simulink library "sm_rollerV_lib_lower_frame_r9"  (R2026a)
settings: Solver=VariableStepAuto
undefined symbols (not defined in the file): Excv, Left, Right
libraries: sm_rollerV_lib_underc_elem x2, sm_rollerV_lib_underc_i1u2l7 x2
Description:
  | Copyright 2023-2026 The MathWorks, Inc.
settings Model: Creator=smiller  LastModifiedBy=smiller

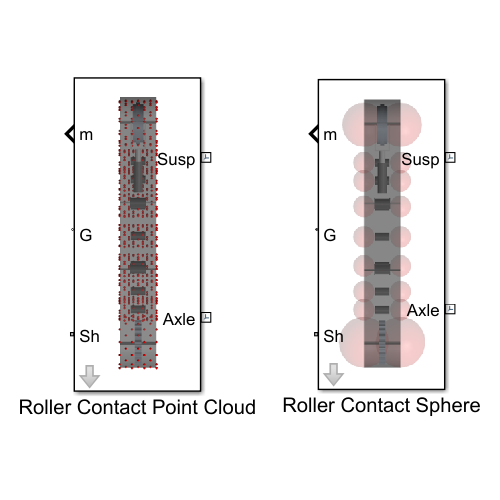
[thumbnail: Simulink's stored preview of the top-level diagram]
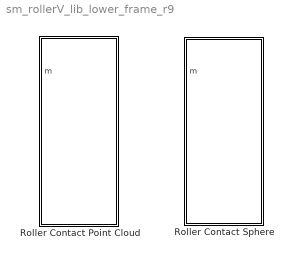
== system sm_rollerV_lib_lower_frame_r9 ==
  Roller Contact Point Cloud : Subsystem  mask(Lower Frame with Roller Point Cloud Contact Geometry){popup_leftOrRight=Left, sprk_xc=Excv.Sprocket.sprocket_xc, sprk_len=Excv.Sprocket.sprk_width, sprk_rho=Excv.Sprocket.density, sprk_clr=Excv.Sprocket.clr, sprk_opc=Excv.Sprocket.opc, sprk_contact_geo_ptcld=Excv.Sprocket.ground_contact.ptcld.pts, sprk_contact_geo_rad=Excv.Sprocket.ground_contact.ptcld.rad, sprk_contact_geo_clr=Excv.Sprocket.ground_contact.ptcld.clr, sprk_contact_geo_opc=Excv.Sprocket.ground_contact.ptcld.opc, idler_rad=Excv.Idler.rad, idler_len=Excv.Idler.len, idler_rho=Excv.Idler.rho, idler_clr=Excv.Idler.clr, idler_opc=Excv.Idler.opc, idler_contact_geo_ptcld=Excv.Idler.ground_contact.ptcld.pts, idler_contact_geo_rad=Excv.Idler.ground_contact.ptcld.rad, idler_contact_geo_clr=Excv.Idler.ground_contact.ptcld.clr, idler_contact_geo_opc=Excv.Idler.ground_contact.ptcld.opc, roller_upper_rad=Excv.Roller.Upper.rad, roller_upper_len=Excv.Roller.Upper.len, roller_upper_rho=Excv.Roller.Upper.rho, roller_upper_clr=Excv.Roller.Upper.clr, roller_upper_opc=Excv.Roller.Upper.opc, roller_upper_contgeo_clr=[1.0 0.0 0.0], roller_upper_contgeo_opc=1, roller_lower_rad=Excv.Roller.Lower.rad, roller_lower_len=Excv.Roller.Lower.len, roller_lower_rho=Excv.Roller.Lower.rho, roller_lower_clr=Excv.Roller.Lower.clr, roller_lower_opc=Excv.Roller.Lower.opc, roller_lower_contgeo_ptcld=Excv.Roller.Lower.ground_contact.ptcld.pts, roller_lower_contgeo_rad=Excv.Roller.Lower.ground_contact.ptcld.rad, roller_lower_contgeo_clr=Excv.Roller.Lower.ground_contact.ptcld.clr, roller_lower_contgeo_opc=Excv.Roller.Lower.ground_contact.ptcld.opc, tensioner_cyl_len=Excv.Idler.Tensioner.cyl.len, tensioner_cyl_rad=Excv.Idler.Tensioner.cyl.rad, tensioner_cyl_rho=Excv.Idler.Tensioner.cyl.rho, tensioner_cyl_clr=Excv.Idler.Tensioner.cyl.clr, tensioner_cyl_opc=Excv.Idler.Tensioner.cyl.opc, tensioner_pist_len=Excv.Idler.Tensioner.piston.len, tensioner_pist_rad=Excv.Idler.Tensioner.piston.rad, tensioner_pist_rho=Excv.Idler.Tensioner.piston.rho, tensioner_pist_clr=Excv.Idler.Tensioner.piston.clr, tensioner_pist_opc=Excv.Idler.Tensioner.piston.opc, tensioner_br_length=Excv.Idler.Tensioner.bracket.len, tensioner_br_width=Excv.Idler.Tensioner.bracket.wid, tensioner_br_height=Excv.Idler.Tensioner.bracket.height, tensioner_br_thk=Excv.Idler.Tensioner.bracket.thk, tensioner_br_rho=Excv.Idler.Tensioner.bracket.rho, tensioner_br_clr=Excv.Idler.Tensioner.bracket.clr, tensioner_br_opc=Excv.Idler.Tensioner.bracket.opc, idler_max_ext=Excv.Idler.Tensioner.cyl.max_ext, sprk_rolling_rad=Excv.Sprocket.ground_contact.rolling_radius, idler_rolling_rad=Excv.Idler.ground_contact.rolling_radius, roller_lower_rolling_rad=Excv.Roller.Lower.ground_contact.rolling_radius, lext=1e-3, track_w=Excv.Shoe.w, sprocket_cyl_clr=Excv.Sprocket.clr, sprocket_cyl_opc=1, idler_cyl_clr=Excv.Idler.clr, idler_cyl_opc=1, roller_cyl_clr=Excv.Roller.Lower.clr, roller_cyl_opc=1, accMn=0.65, accMx=0.75, acc_clr=[0.8 0.8 0.8], acc_opc=1, roller_upper_x=Excv.Frame.Sprk2UpperX, roller_lower_x=Excv.Frame.Sprk2LowerX, idler_x=Excv.Frame.IdlerAssyX, axle_x=Excv.Frame.AxleX, roller_upper_y=Excv.Frame.Sprk2UpperY, roller_lower_y=Excv.Frame.Sprk2LowerY, idler_y=Excv.Frame.Sprk2IdlerY, axle_y=Excv.Frame.AxleY, frame_cg_offset=Excv.Frame.CGOffset, frame_mass=Excv.Frame.Mass, frame_moi=Excv.Frame.MOI, frame_poi=Excv.Frame.POI, frame_susp_offset=Excv.Frame.SuspOffset, track_m=Excv.Vis.Track.m, track_cg_offset=Excv.Vis.Track.cg, track_moi=Excv.Vis.Track.moi, track_poi=Excv.Vis.Track.poi, track_xc=Excv.Vis.Track.track_xc, track_clr=Excv.Vis.Track.clr, track_opc=Excv.Vis.Track.opc, popup_sense_roller=Constraint Force}
      mask prompts: popup_leftOrRight "Left or Right"; sprk_xc "Extrusion Data [x y] (m)"; sprk_len "Length (m)"; sprk_rho "Density (kg/m^3)"; sprk_clr "Color [R G B] (0-1)"; sprk_opc "Opacity (0-1)"; sprk_contact_geo_ptcld "Point Cloud Data [x y z] (m)"; sprk_contact_geo_rad "Radius (m)"; sprk_contact_geo_clr "Color [R G B] (0-1)"; sprk_contact_geo_opc "Opacity (0-1)"; idler_rad "Idler Radius (m)"; idler_len "Length (m)"; idler_rho "Density (kg/m^3)"; idler_clr "Color [R G B] (0-1)"; idler_opc "Opacity (0-1)"; idler_contact_geo_ptcld "Point Cloud Data [x y z] (m)"; idler_contact_geo_rad "Point Radius (m)"; idler_contact_geo_clr "Color [R G B] (0-1)"; idler_contact_geo_opc "Opacity (0-1)"; roller_upper_rad "Radius (m)"; roller_upper_len "Length (m)"; roller_upper_rho "Density (kg/m^3)"; roller_upper_clr "Color [R G B] (0-1)"; roller_upper_opc "Opacity (0-1)"; roller_upper_contgeo_clr "Color [R G B] (0-1)"; roller_upper_contgeo_opc "Opacity (0-1)"; roller_lower_rad "Lower Roller Radius (m)"; roller_lower_len "Length (m)"; roller_lower_rho "Density (kg/m^3)"; roller_lower_clr "Color [R G B] (0-1)"; roller_lower_opc "Opacity (0-1)"; roller_lower_contgeo_ptcld "Point Cloud [x y z] (m)"; roller_lower_contgeo_rad "Point Radius (m)"; roller_lower_contgeo_clr "Color [R G B] (0-1)"; roller_lower_contgeo_opc "Opacity (0-1)"; tensioner_cyl_len "Length (m)"; tensioner_cyl_rad "Radius (m)"; tensioner_cyl_rho "Density (kg/m^3)"; tensioner_cyl_clr "Color [R G B] (0-1)"; tensioner_cyl_opc "Opacity (0-1)"; tensioner_pist_len "Length (m)"; tensioner_pist_rad "Radius (m)"; tensioner_pist_rho "Density (kg/m^3)"; tensioner_pist_clr "Color [R G B] (0-1)"; tensioner_pist_opc "Opacity (0.1)"; tensioner_br_length "Length (m)"; tensioner_br_width "Width (m)"; tensioner_br_height "Height (m)"; tensioner_br_thk "Thickness (m)"; tensioner_br_rho "Density (kg/m^3)"; tensioner_br_clr "Color [R G B] (0-1)"; tensioner_br_opc "Opacity (0-1)"; idler_max_ext "Max Extension in Track (m)"; sprk_rolling_rad "Sprocket Rolling Radius (m)"; idler_rolling_rad "Idler Rolling Radius (m)"; roller_lower_rolling_rad "Lower Roller Rolling Radius (m)"; lext "Length Extensions (m)"; track_w "Shoe Width (m)"; sprocket_cyl_clr "Cylinder Color [R G B] (0-1)"; sprocket_cyl_opc "Cylinder Opacity (0-1)"; idler_cyl_clr "Cylinder Color [R G B] (0-1)"; idler_cyl_opc "Cylinder Opacity (0-1)"; roller_cyl_clr "Cylinder Color [R G B] (0-1)"; roller_cyl_opc "Cylinder Opacity (0-1)"; accMn "Accent Min Radius (0-1)"; accMx "Accent Max Radius (0-1)"; acc_clr "Accent Color [R G B] (0-1)"; acc_opc "Accent Opacity (0-1)"; roller_upper_x "Upper Rollers (vector) (m)"; roller_lower_x "Lower Rollers (vector) (m)"; idler_x "Idler Wheel (m)"; axle_x "Axle Offset (m)"; roller_upper_y "Sprocket to Upper Rollers (m)"; roller_lower_y "Sprocket to Lower Rollers (m)"; idler_y "Sprocket to Idler (m)"; axle_y "Sprocket to Axle (m)"; frame_cg_offset "CG Offset from Sprocket [x y z] (m)"; frame_mass "Mass (kg)"; frame_moi "Moments of Inertia [Ixx Iyy Izz] (kg*m^2)"; frame_poi "Products of Inertia [Ixx Iyy Izz] (kg*m^2)"; frame_susp_offset "Suspension Offset from Sprocket [x y z] (m)"; track_m "Mass"; track_cg_offset "CG Offset from Sprocket Ctr [x y z] (m)"; track_moi "Moments of Inertia  (kg*m^2)"; track_poi "Products of Inertia  (kg*m^2)"; track_xc "Track Visual Extrusion Profile [x y] (m)"; track_clr "Color [R G B] (0-1)"; track_opc "Opacity (0-1)"; popup_sense_roller "Roller"
      mask help: Models an undercarriage with rollers that contact the ground via a point cloud. Includes sprocket, rollers, and idler with tensioner. The sprocket has a 1D rotational mechanical interface to the drivetrain.
      mask init:
      | bh = gcb;
      | set_param([bh '/Undercarriage'],'popup_sense_roller',get_param(bh,'popup_sense_roller'));
      mask TypeOptions popup_leftOrRight: Undercarriage/popup_leftOrRight
      mask TypeOptions sprk_xc: Undercarriage/sprk_xc
      mask TypeOptions sprk_len: Undercarriage/sprk_len
      mask TypeOptions sprk_rho: Undercarriage/sprk_rho
      mask TypeOptions sprk_clr: Undercarriage/sprk_clr
      mask TypeOptions sprk_opc: Undercarriage/sprk_opc
      mask TypeOptions sprk_contact_geo_ptcld: Undercarriage/sprk_contact_geo_ptcld
      mask TypeOptions sprk_contact_geo_rad: Undercarriage/sprk_contact_geo_rad
      mask TypeOptions sprk_contact_geo_clr: Undercarriage/sprk_contact_geo_clr
      mask TypeOptions sprk_contact_geo_opc: Undercarriage/sprk_contact_geo_opc
      mask TypeOptions idler_rad: Undercarriage/idler_rad
      mask TypeOptions idler_len: Undercarriage/idler_len
      mask TypeOptions idler_rho: Undercarriage/idler_rho
      mask TypeOptions idler_clr: Undercarriage/idler_clr
      mask TypeOptions idler_opc: Undercarriage/idler_opc
      mask TypeOptions idler_contact_geo_ptcld: Undercarriage/idler_contact_geo_ptcld
      mask TypeOptions idler_contact_geo_rad: Undercarriage/idler_contact_geo_rad
      mask TypeOptions idler_contact_geo_clr: Undercarriage/idler_contact_geo_clr
      mask TypeOptions idler_contact_geo_opc: Undercarriage/idler_contact_geo_opc
      mask TypeOptions roller_upper_rad: Undercarriage/roller_upper_rad
      mask TypeOptions roller_upper_len: Undercarriage/roller_upper_len
      mask TypeOptions roller_upper_rho: Undercarriage/roller_upper_rho
      mask TypeOptions roller_upper_clr: Undercarriage/roller_upper_clr
      mask TypeOptions roller_upper_opc: Undercarriage/roller_upper_opc
      mask TypeOptions roller_upper_contgeo_clr: Undercarriage/roller_upper_contgeo_clr
      mask TypeOptions roller_upper_contgeo_opc: Undercarriage/roller_upper_contgeo_opc
      mask TypeOptions roller_lower_rad: Undercarriage/roller_lower_rad
      mask TypeOptions roller_lower_len: Undercarriage/roller_lower_len
      mask TypeOptions roller_lower_rho: Undercarriage/roller_lower_rho
      mask TypeOptions roller_lower_clr: Undercarriage/roller_lower_clr
      mask TypeOptions roller_lower_opc: Undercarriage/roller_lower_opc
      mask TypeOptions roller_lower_contgeo_ptcld: Undercarriage/roller_lower_contgeo_ptcld
      mask TypeOptions roller_lower_contgeo_rad: Undercarriage/roller_lower_contgeo_rad
      mask TypeOptions roller_lower_contgeo_clr: Undercarriage/roller_lower_contgeo_clr
      mask TypeOptions roller_lower_contgeo_opc: Undercarriage/roller_lower_contgeo_opc
      mask TypeOptions tensioner_cyl_len: Undercarriage/tensioner_cyl_len
      mask TypeOptions tensioner_cyl_rad: Undercarriage/tensioner_cyl_rad
      mask TypeOptions tensioner_cyl_rho: Undercarriage/tensioner_cyl_rho
      mask TypeOptions tensioner_cyl_clr: Undercarriage/tensioner_cyl_clr
      mask TypeOptions tensioner_cyl_opc: Undercarriage/tensioner_cyl_opc
      mask TypeOptions tensioner_pist_len: Undercarriage/tensioner_pist_len
      mask TypeOptions tensioner_pist_rad: Undercarriage/tensioner_pist_rad
      mask TypeOptions tensioner_pist_rho: Undercarriage/tensioner_pist_rho
      mask TypeOptions tensioner_pist_clr: Undercarriage/tensioner_pist_clr
      mask TypeOptions tensioner_pist_opc: Undercarriage/tensioner_pist_opc
      mask TypeOptions tensioner_br_length: Undercarriage/tensioner_br_length
      mask TypeOptions tensioner_br_width: Undercarriage/tensioner_br_width
      mask TypeOptions tensioner_br_height: Undercarriage/tensioner_br_height
      mask TypeOptions tensioner_br_thk: Undercarriage/tensioner_br_thk
      mask TypeOptions tensioner_br_rho: Undercarriage/tensioner_br_rho
      mask TypeOptions tensioner_br_clr: Undercarriage/tensioner_br_clr
      mask TypeOptions tensioner_br_opc: Undercarriage/tensioner_br_opc
      mask TypeOptions idler_max_ext: Undercarriage/idler_max_ext
      mask TypeOptions sprk_rolling_rad: Undercarriage/sprk_rolling_rad
      mask TypeOptions idler_rolling_rad: Undercarriage/idler_rolling_rad
      mask TypeOptions roller_lower_rolling_rad: Undercarriage/roller_lower_rolling_rad
      mask TypeOptions lext: Undercarriage/lext
      mask TypeOptions track_w: Track/track_w | Undercarriage/cyl_len
      mask TypeOptions sprocket_cyl_clr: Undercarriage/sprocket_cyl_clr
      mask TypeOptions sprocket_cyl_opc: Undercarriage/sprocket_cyl_opc
      mask TypeOptions idler_cyl_clr: Undercarriage/idler_cyl_clr
      mask TypeOptions idler_cyl_opc: Undercarriage/idler_cyl_opc
      mask TypeOptions roller_cyl_clr: Undercarriage/roller_cyl_clr
      mask TypeOptions roller_cyl_opc: Undercarriage/roller_cyl_opc
      mask TypeOptions accMn: Undercarriage/accMn
      mask TypeOptions accMx: Undercarriage/accMx
      mask TypeOptions acc_clr: Undercarriage/acc_clr
      mask TypeOptions acc_opc: Undercarriage/acc_opc
      mask TypeOptions roller_upper_x: Undercarriage/roller_upper_x
      mask TypeOptions roller_lower_x: Undercarriage/roller_lower_x
      mask TypeOptions idler_x: Undercarriage/idler_x
      mask TypeOptions axle_x: Track/track_axle_offset_x | Undercarriage/axle_x
      mask TypeOptions roller_upper_y: Undercarriage/roller_upper_y
      mask TypeOptions roller_lower_y: Undercarriage/roller_lower_y
      mask TypeOptions idler_y: Undercarriage/idler_y
      mask TypeOptions axle_y: Track/track_axle_offset_y | Undercarriage/axle_y
      mask TypeOptions frame_cg_offset: Undercarriage/frame_cg_offset
      mask TypeOptions frame_mass: Undercarriage/frame_mass
      mask TypeOptions frame_moi: Undercarriage/frame_moi
      mask TypeOptions frame_poi: Undercarriage/frame_poi
      mask TypeOptions frame_susp_offset: Undercarriage/frame_susp_offset
      mask TypeOptions track_m: Track/track_m
      mask TypeOptions track_cg_offset: Track/track_cg_offset
      mask TypeOptions track_moi: Track/track_moi
      mask TypeOptions track_poi: Track/track_poi
      mask TypeOptions track_xc: Track/track_xc
      mask TypeOptions track_clr: Track/track_clr
      mask TypeOptions track_opc: Track/track_opc
      mask TypeOptions popup_sense_roller: Constraint Force | Actuator Torque
      mask DialogControl cont_sprocket Prompt: Sprocket
      mask DialogControl cont_sprocket_solid Prompt: Solid
      mask DialogControl cont_sprocket_contact_geo Prompt: Contact Geometry
      mask DialogControl cont_idler Prompt: Idler
      mask DialogControl cont_idler_solid Prompt: Solid
      mask DialogControl cont_idler_contact_geo Prompt: Contact Geometry
      mask DialogControl cont_rollers Prompt: Rollers
      mask DialogControl cont_roller_upper Prompt: Upper
      mask DialogControl cont_rollers_upper_contact_geo Prompt: Contact Geometry
      mask DialogControl cont_rollers_lower Prompt: Lower
      mask DialogControl cont_rollers_lower_contact_geo Prompt: Contact Geometry
      mask DialogControl cont_tensioner Prompt: Tensioner
      mask DialogControl cont_tensioner_cyl Prompt: Cylinder
      mask DialogControl cont_tensioner_pist Prompt: Piston
      mask DialogControl cont_tensioner_brkt Prompt: Bracket
      mask DialogControl cont_tensioner_assembly Prompt: Assembly
      mask DialogControl cont_rolling Prompt: Rolling
      mask DialogControl cont_constr_len Prompt: Constraints and Length
      mask DialogControl cont_rollvis_sprk Prompt: Roller Visual: Sprocket
      mask DialogControl cont_rollvis_idler Prompt: Roller Visual: Idler
      mask DialogControl cont_rollvis_roller Prompt: Roller Visual: Roller
      mask DialogControl cont_accvis Prompt: Accent Visual
      mask DialogControl cont_frame Prompt: Frame
      mask DialogControl cont_offset_x Prompt: Longitudinal Offsets from Sprocket
      mask DialogControl cont_offset_y Prompt: Vertical Offsets
      mask DialogControl cont_mass Prompt: Mass and Inertia
      mask DialogControl cont_susp Prompt: Suspension Offset
      mask DialogControl cont_track Prompt: Track
      mask DialogControl cont_sensing Prompt: Sensing
      mask Display: image('sm_excv_track_rollerptcld_topview_IMAGE.png');
  Roller Contact Sphere : Subsystem  mask(Lower Frame with Roller Sphere Contact Geometry){popup_leftOrRight=Right, sprk_xc=Excv.Sprocket.sprocket_xc, sprk_len=Excv.Sprocket.sprk_width, sprk_rho=Excv.Sprocket.density, sprk_clr=Excv.Sprocket.clr, sprk_opc=Excv.Sprocket.opc, sprk_contact_geo_clr=Excv.Sprocket.ground_contact.sphere.clr, sprk_contact_geo_opc=Excv.Sprocket.ground_contact.sphere.opc, idler_rad=Excv.Idler.rad, idler_len=Excv.Idler.len, idler_rho=Excv.Idler.rho, idler_clr=Excv.Idler.clr, idler_opc=Excv.Idler.opc, idler_contact_geo_clr=Excv.Idler.ground_contact.sphere.clr, idler_contact_geo_opc=Excv.Idler.ground_contact.sphere.opc, roller_upper_rad=Excv.Roller.Upper.rad, roller_upper_len=Excv.Roller.Upper.len, roller_upper_rho=Excv.Roller.Upper.rho, roller_upper_clr=Excv.Roller.Upper.clr, roller_upper_opc=Excv.Roller.Upper.opc, roller_upper_contgeo_clr=[1.0 0.0 0.0], roller_upper_contgeo_opc=1, roller_lower_rad=Excv.Roller.Lower.rad, roller_lower_len=Excv.Roller.Lower.len, roller_lower_rho=Excv.Roller.Lower.rho, roller_lower_clr=Excv.Roller.Lower.clr, roller_lower_opc=Excv.Roller.Lower.opc, roller_lower_contgeo_clr=Excv.Roller.Lower.ground_contact.sphere.clr, roller_lower_contgeo_opc=Excv.Roller.Lower.ground_contact.sphere.opc, tensioner_cyl_len=Excv.Idler.Tensioner.cyl.len, tensioner_cyl_rad=Excv.Idler.Tensioner.cyl.rad, tensioner_cyl_rho=Excv.Idler.Tensioner.cyl.rho, tensioner_cyl_clr=Excv.Idler.Tensioner.cyl.clr, tensioner_cyl_opc=Excv.Idler.Tensioner.cyl.opc, tensioner_pist_len=Excv.Idler.Tensioner.piston.len, tensioner_pist_rad=Excv.Idler.Tensioner.piston.rad, tensioner_pist_rho=Excv.Idler.Tensioner.piston.rho, tensioner_pist_clr=Excv.Idler.Tensioner.piston.clr, tensioner_pist_opc=Excv.Idler.Tensioner.piston.opc, tensioner_br_length=Excv.Idler.Tensioner.bracket.len, tensioner_br_width=Excv.Idler.Tensioner.bracket.wid, tensioner_br_height=Excv.Idler.Tensioner.bracket.height, tensioner_br_thk=Excv.Idler.Tensioner.bracket.thk, tensioner_br_rho=Excv.Idler.Tensioner.bracket.rho, tensioner_br_clr=Excv.Idler.Tensioner.bracket.clr, tensioner_br_opc=Excv.Idler.Tensioner.bracket.opc, idler_max_ext=Excv.Idler.Tensioner.cyl.max_ext, sprk_rolling_rad=Excv.Sprocket.ground_contact.rolling_radius, idler_rolling_rad=Excv.Idler.ground_contact.rolling_radius, roller_lower_rolling_rad=Excv.Roller.Lower.ground_contact.rolling_radius, track_w=Excv.Shoe.w, roller_upper_x=Excv.Frame.Sprk2UpperX, roller_lower_x=Excv.Frame.Sprk2LowerX, idler_x=Excv.Frame.IdlerAssyX, axle_x=Excv.Frame.AxleX, roller_upper_y=Excv.Frame.Sprk2UpperY, roller_lower_y=Excv.Frame.Sprk2LowerY, idler_y=Excv.Frame.Sprk2IdlerY, axle_y=Excv.Frame.AxleY, frame_cg_offset=Excv.Frame.CGOffset, frame_mass=Excv.Frame.Mass, frame_moi=Excv.Frame.MOI, frame_poi=Excv.Frame.POI, frame_susp_offset=Excv.Frame.SuspOffset, track_m=Excv.Vis.Track.m, track_cg_offset=Excv.Vis.Track.cg, track_moi=Excv.Vis.Track.moi, track_poi=Excv.Vis.Track.poi, track_xc=Excv.Vis.Track.track_xc, track_clr=Excv.Vis.Track.clr, track_opc=Excv.Vis.Track.opc, popup_sense_roller=Actuator Torque}
      mask prompts: popup_leftOrRight "Left or Right"; sprk_xc "Extrusion Data [x y] (m)"; sprk_len "Length (m)"; sprk_rho "Density (kg/m^3)"; sprk_clr "Color [R G B] (0-1)"; sprk_opc "Opacity (0-1)"; sprk_contact_geo_clr "Color [R G B] (0-1)"; sprk_contact_geo_opc "Opacity (0-1)"; idler_rad "Idler Radius (m)"; idler_len "Length (m)"; idler_rho "Density (kg/m^3)"; idler_clr "Color [R G B] (0-1)"; idler_opc "Opacity (0-1)"; idler_contact_geo_clr "Color [R G B] (0-1)"; idler_contact_geo_opc "Opacity (0-1)"; roller_upper_rad "Radius (m)"; roller_upper_len "Length (m)"; roller_upper_rho "Density (kg/m^3)"; roller_upper_clr "Color [R G B] (0-1)"; roller_upper_opc "Opacity (0-1)"; roller_upper_contgeo_clr "Color [R G B] (0-1)"; roller_upper_contgeo_opc "Opacity (0-1)"; roller_lower_rad "Lower Roller Radius (m)"; roller_lower_len "Length (m)"; roller_lower_rho "Density (kg/m^3)"; roller_lower_clr "Color [R G B] (0-1)"; roller_lower_opc "Opacity (0-1)"; roller_lower_contgeo_clr "Color [R G B] (0-1)"; roller_lower_contgeo_opc "Opacity (0-1)"; tensioner_cyl_len "Length (m)"; tensioner_cyl_rad "Radius (m)"; tensioner_cyl_rho "Density (kg/m^3)"; tensioner_cyl_clr "Color [R G B] (0-1)"; tensioner_cyl_opc "Opacity (0-1)"; tensioner_pist_len "Length (m)"; tensioner_pist_rad "Radius (m)"; tensioner_pist_rho "Density (kg/m^3)"; tensioner_pist_clr "Color [R G B] (0-1)"; tensioner_pist_opc "Opacity (0.1)"; tensioner_br_length "Length (m)"; tensioner_br_width "Width (m)"; tensioner_br_height "Height (m)"; tensioner_br_thk "Thickness (m)"; tensioner_br_rho "Density (kg/m^3)"; tensioner_br_clr "Color [R G B] (0-1)"; tensioner_br_opc "Opacity (0-1)"; idler_max_ext "Max Extension in Track (m)"; sprk_rolling_rad "Sprocket Rolling Radius (m)"; idler_rolling_rad "Idler Rolling Radius (m)"; roller_lower_rolling_rad "Lower Roller Rolling Radius (m)"; track_w "Track Visual Extrusion Length [(m)"; roller_upper_x "Upper Rollers (vector) (m)"; roller_lower_x "Lower Rollers (vector) (m)"; idler_x "Idler Wheel (m)"; axle_x "Axle Offset (m)"; roller_upper_y "Sprocket to Upper Rollers (m)"; roller_lower_y "Sprocket to Lower Rollers (m)"; idler_y "Sprocket to Idler (m)"; axle_y "Sprocket to Axle (m)"; frame_cg_offset "CG Offset from Sprocket [x y z] (m)"; frame_mass "Mass (kg)"; frame_moi "Moments of Inertia [Ixx Iyy Izz] (kg*m^2)"; frame_poi "Products of Inertia [Ixx Iyy Izz] (kg*m^2)"; frame_susp_offset "Suspension Offset from Sprocket [x y z] (m)"; track_m "Mass"; track_cg_offset "CG Offset from Sprocket Ctr [x y z] (m)"; track_moi "Moments of Inertia  (kg*m^2)"; track_poi "Products of Inertia  (kg*m^2)"; track_xc "Track Visual Extrusion Profile [x y] (m)"; track_clr "Color [R G B] (0-1)"; track_opc "Opacity (0-1)"; popup_sense_roller "Roller"
      mask help: Models an undercrariage with rollers that contact the ground via spheres. Includes sprocket, rollers, and idler with tensioner. The sprocket has a 1D rotational mechanical interface to the drivetrain.
      mask TypeOptions popup_leftOrRight: Undercarriage/popup_leftOrRight
      mask TypeOptions sprk_xc: Undercarriage/sprk_xc
      mask TypeOptions sprk_len: Undercarriage/sprk_len
      mask TypeOptions sprk_rho: Undercarriage/sprk_rho
      mask TypeOptions sprk_clr: Undercarriage/sprk_clr
      mask TypeOptions sprk_opc: Undercarriage/sprk_opc
      mask TypeOptions sprk_contact_geo_clr: Undercarriage/sprk_contact_geo_clr
      mask TypeOptions sprk_contact_geo_opc: Undercarriage/sprk_contact_geo_opc
      mask TypeOptions idler_rad: Undercarriage/idler_rad
      mask TypeOptions idler_len: Undercarriage/idler_len
      mask TypeOptions idler_rho: Undercarriage/idler_rho
      mask TypeOptions idler_clr: Undercarriage/idler_clr
      mask TypeOptions idler_opc: Undercarriage/idler_opc
      mask TypeOptions idler_contact_geo_clr: Undercarriage/idler_contact_geo_clr
      mask TypeOptions idler_contact_geo_opc: Undercarriage/idler_contact_geo_opc
      mask TypeOptions roller_upper_rad: Undercarriage/roller_upper_rad
      mask TypeOptions roller_upper_len: Undercarriage/roller_upper_len
      mask TypeOptions roller_upper_rho: Undercarriage/roller_upper_rho
      mask TypeOptions roller_upper_clr: Undercarriage/roller_upper_clr
      mask TypeOptions roller_upper_opc: Undercarriage/roller_upper_opc
      mask TypeOptions roller_upper_contgeo_clr: Undercarriage/roller_upper_contgeo_clr
      mask TypeOptions roller_upper_contgeo_opc: Undercarriage/roller_upper_contgeo_opc
      mask TypeOptions roller_lower_rad: Undercarriage/roller_lower_rad
      mask TypeOptions roller_lower_len: Undercarriage/roller_lower_len
      mask TypeOptions roller_lower_rho: Undercarriage/roller_lower_rho
      mask TypeOptions roller_lower_clr: Undercarriage/roller_lower_clr
      mask TypeOptions roller_lower_opc: Undercarriage/roller_lower_opc
      mask TypeOptions roller_lower_contgeo_clr: Undercarriage/roller_lower_contgeo_clr
      mask TypeOptions roller_lower_contgeo_opc: Undercarriage/roller_lower_contgeo_opc
      mask TypeOptions tensioner_cyl_len: Undercarriage/tensioner_cyl_len
      mask TypeOptions tensioner_cyl_rad: Undercarriage/tensioner_cyl_rad
      mask TypeOptions tensioner_cyl_rho: Undercarriage/tensioner_cyl_rho
      mask TypeOptions tensioner_cyl_clr: Undercarriage/tensioner_cyl_clr
      mask TypeOptions tensioner_cyl_opc: Undercarriage/tensioner_cyl_opc
      mask TypeOptions tensioner_pist_len: Undercarriage/tensioner_pist_len
      mask TypeOptions tensioner_pist_rad: Undercarriage/tensioner_pist_rad
      mask TypeOptions tensioner_pist_rho: Undercarriage/tensioner_pist_rho
      mask TypeOptions tensioner_pist_clr: Undercarriage/tensioner_pist_clr
      mask TypeOptions tensioner_pist_opc: Undercarriage/tensioner_pist_opc
      mask TypeOptions tensioner_br_length: Undercarriage/tensioner_br_length
      mask TypeOptions tensioner_br_width: Undercarriage/tensioner_br_width
      mask TypeOptions tensioner_br_height: Undercarriage/tensioner_br_height
      mask TypeOptions tensioner_br_thk: Undercarriage/tensioner_br_thk
      mask TypeOptions tensioner_br_rho: Undercarriage/tensioner_br_rho
      mask TypeOptions tensioner_br_clr: Undercarriage/tensioner_br_clr
      mask TypeOptions tensioner_br_opc: Undercarriage/tensioner_br_opc
      mask TypeOptions idler_max_ext: Undercarriage/idler_max_ext
      mask TypeOptions sprk_rolling_rad: Undercarriage/sprk_rolling_rad
      mask TypeOptions idler_rolling_rad: Undercarriage/idler_rolling_rad
      mask TypeOptions roller_lower_rolling_rad: Undercarriage/roller_lower_rolling_rad
      mask TypeOptions track_w: Track/track_w | Undercarriage/shoe_w
      mask TypeOptions roller_upper_x: Undercarriage/roller_upper_x
      mask TypeOptions roller_lower_x: Undercarriage/roller_lower_x
      mask TypeOptions idler_x: Undercarriage/idler_x
      mask TypeOptions axle_x: Track/track_axle_offset_x | Undercarriage/axle_x
      mask TypeOptions roller_upper_y: Undercarriage/roller_upper_y
      mask TypeOptions roller_lower_y: Undercarriage/roller_lower_y
      mask TypeOptions idler_y: Undercarriage/idler_y
      mask TypeOptions axle_y: Track/track_axle_offset_y | Undercarriage/axle_y
      mask TypeOptions frame_cg_offset: Undercarriage/frame_cg_offset
      mask TypeOptions frame_mass: Undercarriage/frame_mass
      mask TypeOptions frame_moi: Undercarriage/frame_moi
      mask TypeOptions frame_poi: Undercarriage/frame_poi
      mask TypeOptions frame_susp_offset: Undercarriage/frame_susp_offset
      mask TypeOptions track_m: Track/track_m
      mask TypeOptions track_cg_offset: Track/track_cg_offset
      mask TypeOptions track_moi: Track/track_moi
      mask TypeOptions track_poi: Track/track_poi
      mask TypeOptions track_xc: Track/track_xc
      mask TypeOptions track_clr: Track/track_clr
      mask TypeOptions track_opc: Track/track_opc
      mask TypeOptions popup_sense_roller: Undercarriage/popup_sense_roller
      mask DialogControl cont_sprocket Prompt: Sprocket
      mask DialogControl cont_sprocket_solid Prompt: Solid
      mask DialogControl cont_sprocket_contact_geo Prompt: Contact Geometry
      mask DialogControl cont_idler Prompt: Idler
      mask DialogControl cont_idler_solid Prompt: Solid
      mask DialogControl cont_idler_contact_geo Prompt: Contact Geometry
      mask DialogControl cont_rollers Prompt: Rollers
      mask DialogControl cont_roller_upper Prompt: Upper
      mask DialogControl cont_rollers_upper_contact_geo Prompt: Contact Geometry
      mask DialogControl cont_rollers_lower Prompt: Lower
      mask DialogControl cont_rollers_lower_contact_geo Prompt: Contact Geometry
      mask DialogControl cont_tensioner Prompt: Tensioner
      mask DialogControl cont_tensioner_cyl Prompt: Cylinder
      mask DialogControl cont_tensioner_pist Prompt: Piston
      mask DialogControl cont_tensioner_brkt Prompt: Bracket
      mask DialogControl cont_tensioner_assembly Prompt: Assembly
      mask DialogControl cont_rolling Prompt: Rolling
      mask DialogControl cont_const_len Prompt: Constraints and Length
      mask DialogControl cont_frame Prompt: Frame
      mask DialogControl cont_offset_x Prompt: Longitudinal Offsets from Sprocket
      mask DialogControl cont_offset_y Prompt: Vertical Offsets
      mask DialogControl cont_mass Prompt: Mass and Inertia
      mask DialogControl cont_susp Prompt: Suspension Offset
      mask DialogControl cont_track Prompt: Track
      mask DialogControl cont_sensing Prompt: Sensing
      mask Display: image('sm_excv_track_rollersphere_topview_IMAGE.png');

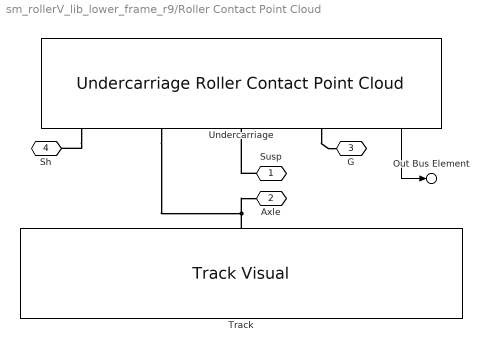
== system sm_rollerV_lib_lower_frame_r9/Roller Contact Point Cloud ==
  Track : sm_rollerV_lib_underc_elem/Track Visual  track_m=track_m  track_cg_offset=track_cg_offset  track_axle_offset_x=axle_x  track_axle_offset_y=axle_y  track_moi=track_moi  track_poi=track_poi  track_xc=track_xc  track_w=track_w  track_clr=track_clr  track_opc=track_opc
  Undercarriage : sm_rollerV_lib_underc_i1u2l7/Undercarriage Roller Contact Point Cloud  popup_leftOrRight=Left  sprk_xc=sprk_xc  sprk_len=sprk_len  sprk_rho=sprk_rho  sprk_clr=sprk_clr  sprk_opc=sprk_opc  sprk_contact_geo_ptcld=sprk_contact_geo_ptcld  sprk_contact_geo_rad=sprk_contact_geo_rad  sprk_contact_geo_clr=sprk_contact_geo_clr  sprk_contact_geo_opc=sprk_contact_geo_opc  idler_rad=idler_rad  idler_len=idler_len  idler_rho=idler_rho  idler_clr=idler_clr  idler_opc=idler_opc  idler_contact_geo_ptcld=idler_contact_geo_ptcld  idler_contact_geo_rad=idler_contact_geo_rad  idler_contact_geo_clr=idler_contact_geo_clr  idler_contact_geo_opc=idler_contact_geo_opc  roller_upper_rad=roller_upper_rad  roller_upper_len=roller_upper_len  roller_upper_rho=roller_upper_rho  roller_upper_clr=roller_upper_clr  roller_upper_opc=roller_upper_opc  roller_upper_contgeo_clr=roller_upper_contgeo_clr  roller_upper_contgeo_opc=roller_upper_contgeo_opc  roller_lower_rad=roller_lower_rad  roller_lower_len=roller_lower_len  roller_lower_rho=roller_lower_rho  roller_lower_clr=roller_lower_clr  roller_lower_opc=roller_lower_opc  roller_lower_contgeo_ptcld=roller_lower_contgeo_ptcld  roller_lower_contgeo_rad=roller_lower_contgeo_rad  roller_lower_contgeo_clr=roller_lower_contgeo_clr  roller_lower_contgeo_opc=roller_lower_contgeo_opc  tensioner_cyl_len=tensioner_cyl_len  tensioner_cyl_rad=tensioner_cyl_rad  tensioner_cyl_rho=tensioner_cyl_rho  tensioner_cyl_clr=tensioner_cyl_clr  tensioner_cyl_opc=tensioner_cyl_opc  tensioner_pist_len=tensioner_pist_len  tensioner_pist_rad=tensioner_pist_rad  tensioner_pist_rho=tensioner_pist_rho  tensioner_pist_clr=tensioner_pist_clr  tensioner_pist_opc=tensioner_pist_opc  tensioner_br_length=tensioner_br_length  tensioner_br_width=tensioner_br_width  tensioner_br_height=tensioner_br_height  tensioner_br_thk=tensioner_br_thk  tensioner_br_rho=tensioner_br_rho  tensioner_br_clr=tensioner_br_clr  tensioner_br_opc=tensioner_br_opc  idler_max_ext=idler_max_ext  sprk_rolling_rad=sprk_rolling_rad  idler_rolling_rad=idler_rolling_rad  roller_lower_rolling_rad=roller_lower_rolling_rad  cyl_len=track_w  lext=lext  roller_cyl_clr=roller_cyl_clr  roller_cyl_opc=roller_cyl_opc  sprocket_cyl_clr=sprocket_cyl_clr  sprocket_cyl_opc=sprocket_cyl_opc  idler_cyl_clr=idler_cyl_clr  idler_cyl_opc=idler_cyl_opc  accMn=accMn  accMx=accMx  acc_clr=acc_clr  acc_opc=acc_opc  roller_upper_x=roller_upper_x  roller_lower_x=roller_lower_x  idler_x=idler_x  axle_x=axle_x  roller_upper_y=roller_upper_y  roller_lower_y=roller_lower_y  idler_y=idler_y  axle_y=axle_y  frame_cg_offset=frame_cg_offset  frame_mass=frame_mass  frame_moi=frame_moi  frame_poi=frame_poi  frame_susp_offset=frame_susp_offset  popup_sense_roller=Constraint Force
      settings: LibrarySourceBlock=|
      | sm_excv_underc_lib/Undercarriage
      | Roller Ground
      | Contact
  Susp : PMIOPort  Side=Left
  Axle : PMIOPort  Port=2  Side=Left
  G : PMIOPort  Port=3  Side=Right
  Sh : PMIOPort  Port=4  Side=Right
  Out Bus Element : Outport  PortName=m  Element=Underc
  wires:
  Undercarriage/1 -> Out Bus Element/1
  connections:
  Track/LConn1 -- Axle/RConn1 -- Undercarriage/RConn3
  Undercarriage/RConn1 -- G/RConn1
  Undercarriage/RConn4 -- Sh/RConn1
  Susp/RConn1 -- Undercarriage/RConn2

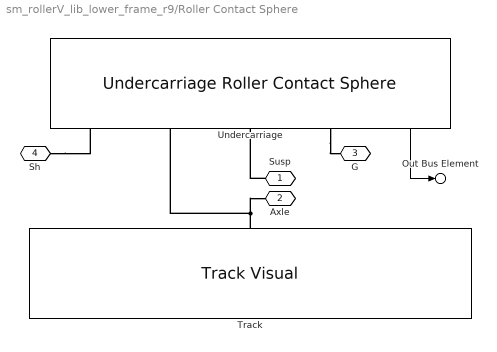
== system sm_rollerV_lib_lower_frame_r9/Roller Contact Sphere ==
  Track : sm_rollerV_lib_underc_elem/Track Visual  track_m=track_m  track_cg_offset=track_cg_offset  track_axle_offset_x=axle_x  track_axle_offset_y=axle_y  track_moi=track_moi  track_poi=track_poi  track_xc=track_xc  track_w=track_w  track_clr=track_clr  track_opc=track_opc
  Undercarriage : sm_rollerV_lib_underc_i1u2l7/Undercarriage Roller Contact Sphere  popup_leftOrRight=Right  sprk_xc=sprk_xc  sprk_len=sprk_len  sprk_rho=sprk_rho  sprk_clr=sprk_clr  sprk_opc=sprk_opc  sprk_contact_geo_clr=sprk_contact_geo_clr  sprk_contact_geo_opc=sprk_contact_geo_opc  idler_rad=idler_rad  idler_len=idler_len  idler_rho=idler_rho  idler_clr=idler_clr  idler_opc=idler_opc  idler_contact_geo_clr=idler_contact_geo_clr  idler_contact_geo_opc=idler_contact_geo_opc  roller_upper_rad=roller_upper_rad  roller_upper_len=roller_upper_len  roller_upper_rho=roller_upper_rho  roller_upper_clr=roller_upper_clr  roller_upper_opc=roller_upper_opc  roller_upper_contgeo_clr=roller_upper_contgeo_clr  roller_upper_contgeo_opc=roller_upper_contgeo_opc  roller_lower_rad=roller_lower_rad  roller_lower_len=roller_lower_len  roller_lower_rho=roller_lower_rho  roller_lower_clr=roller_lower_clr  roller_lower_opc=roller_lower_opc  roller_lower_contgeo_clr=roller_lower_contgeo_clr  roller_lower_contgeo_opc=roller_lower_contgeo_opc  tensioner_cyl_len=tensioner_cyl_len  tensioner_cyl_rad=tensioner_cyl_rad  tensioner_cyl_rho=tensioner_cyl_rho  tensioner_cyl_clr=tensioner_cyl_clr  tensioner_cyl_opc=tensioner_cyl_opc  tensioner_pist_len=tensioner_pist_len  tensioner_pist_rad=tensioner_pist_rad  tensioner_pist_rho=tensioner_pist_rho  tensioner_pist_clr=tensioner_pist_clr  tensioner_pist_opc=tensioner_pist_opc  tensioner_br_length=tensioner_br_length  tensioner_br_width=tensioner_br_width  tensioner_br_height=tensioner_br_height  tensioner_br_thk=tensioner_br_thk  tensioner_br_rho=tensioner_br_rho  tensioner_br_clr=tensioner_br_clr  tensioner_br_opc=tensioner_br_opc  idler_max_ext=idler_max_ext  sprk_rolling_rad=sprk_rolling_rad  idler_rolling_rad=idler_rolling_rad  roller_lower_rolling_rad=roller_lower_rolling_rad  shoe_w=track_w  roller_upper_x=roller_upper_x  roller_lower_x=roller_lower_x  idler_x=idler_x  axle_x=axle_x  roller_upper_y=roller_upper_y  roller_lower_y=roller_lower_y  idler_y=idler_y  axle_y=axle_y  frame_cg_offset=frame_cg_offset  frame_mass=frame_mass  frame_moi=frame_moi  frame_poi=frame_poi  frame_susp_offset=frame_susp_offset  popup_sense_roller=Actuator Torque
      settings: LibrarySourceBlock=|
      | sm_excv_underc_lib/Undercarriage
      | Roller Ground
      | Sphere Contact
  Susp : PMIOPort  Side=Left
  Axle : PMIOPort  Port=2  Side=Left
  G : PMIOPort  Port=3  Side=Right
  Sh : PMIOPort  Port=4  Side=Right
  Out Bus Element : Outport  PortName=m  Element=Underc
  wires:
  Undercarriage/1 -> Out Bus Element/1
  connections:
  Undercarriage/RConn1 -- G/RConn1
  Track/LConn1 -- Axle/RConn1 -- Undercarriage/RConn3
  Sh/RConn1 -- Undercarriage/RConn4
  Susp/RConn1 -- Undercarriage/RConn2
